simulink model "dummy_joint_1"  (R2024b)
settings: Solver=FixedStepAuto  StartTime=0.0  StopTime=10.0  FixedStep=0.001  RelTol=1e-3
libraries: simulink x1
settings Model: Creator=giang  LastModifiedBy=giangnguyen

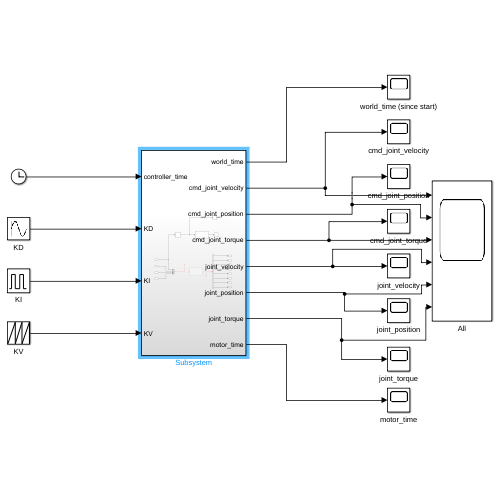
[thumbnail: Simulink's stored preview of the top-level diagram]
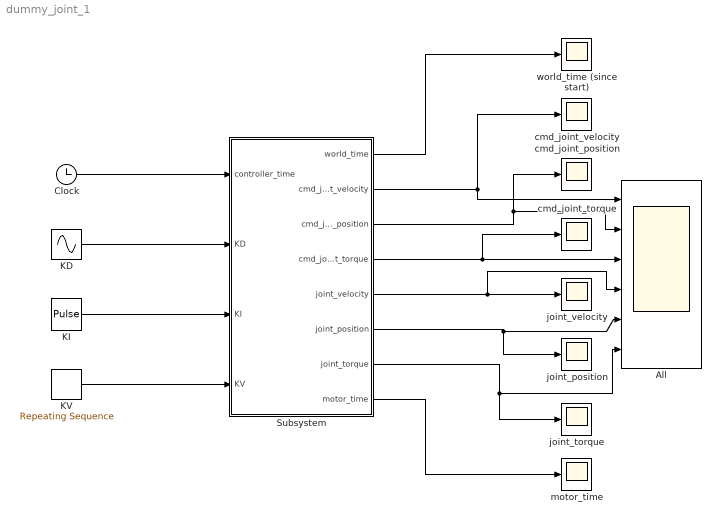
== system dummy_joint_1 ==
  All : Scope  NumInputPorts=6
  Clock : Clock
  KD : Sin  Amplitude=[1]  SampleTime=0
  KI : DiscretePulseGenerator  PulseType=Time based  Period=1  PulseWidth=50
  KV : simulink/Sources/Repeating Sequence  rep_seq_t=[0 2]  rep_seq_y=[0 2]
  Subsystem : Subsystem
  cmd_joint_position : Scope
  cmd_joint_torque : Scope
  cmd_joint_velocity : Scope
  joint_position : Scope
  joint_torque : Scope
  joint_velocity : Scope
  motor_time : Scope
  world_time (since start) : Scope
  wires:
  KD/1 -> Subsystem/2(KD)
  KI/1 -> Subsystem/3(KI)
  KV/1 -> Subsystem/4(KV)
  Subsystem/8(motor_time) -> motor_time/1
  Subsystem/1(world_time) -> world_time (since start)/1
  Subsystem/2(cmd_joint_velocity) -> cmd_joint_velocity/1, All/1
  Subsystem/3(cmd_joint_position) -> cmd_joint_position/1, All/2
  Subsystem/4(cmd_joint_torque) -> cmd_joint_torque/1, All/3
  Subsystem/5(joint_velocity) -> All/4, joint_velocity/1
  Subsystem/6(joint_position) -> joint_position/1, All/5
  Subsystem/7(joint_torque) -> joint_torque/1, All/6
  Clock/1 -> Subsystem/1(controller_time)

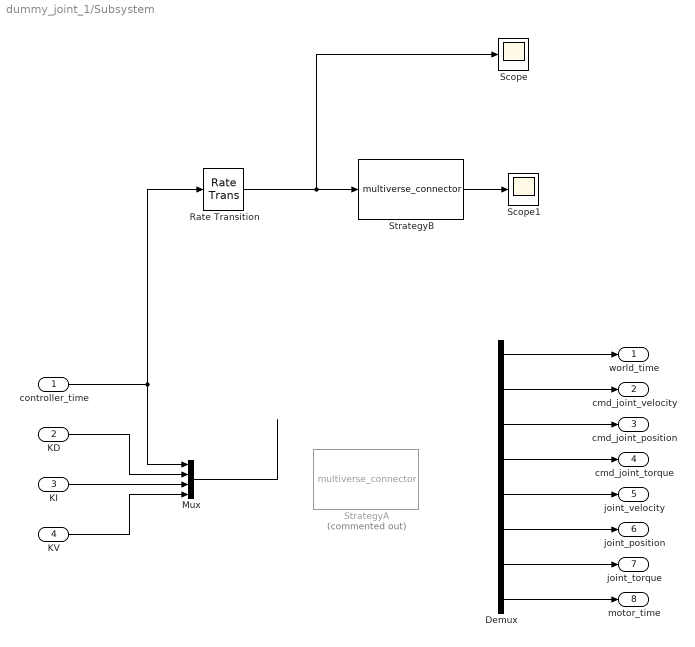
== system dummy_joint_1/Subsystem ==
  controller_time : Inport
  KD : Inport  Port=2
  KI : Inport  Port=3
  KV : Inport  Port=4
  Demux : Demux  Outputs=8
  Mux : Mux
  Rate Transition : RateTransition  OutPortSampleTime=1
  Scope : Scope
  Scope1 : Scope
  StrategyA : S-Function  Commented=on  FunctionName=multiverse_connector  Parameters="'tcp://127.0.0.1' '7000' '7593' 'world' 'matlab_A' '{\"send\": {\"KD\": [\"scalar\"], \"KV\": [\"scalar\"], \"KI\": [\"scalar\"]}, \"receive\": {\"joint_1\": [\"cmd_joint_torque\", \"cmd_joint_angular_velocity\", \"cmd_joint_rvalue\", \"joint_rvalue\", \"joint_angular_velocity\", \"joint_torque\", \"time\"]}}'"  SFunctionDeploymentMode=off  EnableBusSupport=off
  StrategyB : S-Function  FunctionName=multiverse_connector  Parameters="'tcp://127.0.0.1' '7000' '9375' 'world' 'matlab_B' '{\"api_callbacks\": {\"joint_1_simulation\": [{\"get_everything\": [\"1000\"]}]}}}' 1.0"  SFunctionDeploymentMode=off  EnableBusSupport=off
  world_time : Outport
  cmd_joint_velocity : Outport  Port=2
  cmd_joint_position : Outport  Port=3
  cmd_joint_torque : Outport  Port=4
  joint_velocity : Outport  Port=5
  joint_position : Outport  Port=6
  joint_torque : Outport  Port=7
  motor_time : Outport  Port=8
  wires:
  Mux/1 -> ?
  ? -> Demux/1
  Demux/1 -> world_time/1
  Demux/2 -> cmd_joint_velocity/1
  Demux/3 -> cmd_joint_position/1
  Demux/4 -> cmd_joint_torque/1
  Demux/5 -> joint_velocity/1
  Demux/6 -> joint_position/1
  Demux/7 -> joint_torque/1
  Demux/8 -> motor_time/1
  KI/1 -> Mux/3
  KD/1 -> Mux/2
  KV/1 -> Mux/4
  controller_time/1 -> Rate Transition/1, Mux/1
  Rate Transition/1 -> Scope/1, StrategyB/1
  StrategyB/1 -> Scope1/1
